simulink model "BPSK"  (R2024b)
settings: Solver=VariableStepAuto  StartTime=0.0  StopTime=10.0  RelTol=1e-3
undefined symbols (not defined in the file or in its folder): comm, constellation
libraries: commdigbbndpm3 x2, commchan3 x1, commutil2 x1, commsink2 x1, commrflib2 x1, commrandsrc3 x1
settings Model: Creator=sarriola  LastModifiedBy=romaf41
settings SolverCC: AlgebraicLoopSolver=TrustRegion
settings DataIOCC: ReturnWorkspaceOutputs=off
settings DebuggingCC: UnconnectedInputMsg=warning  UnconnectedOutputMsg=warning  UnconnectedLineMsg=warning  ArithmeticOperatorsInVariantConditions=warning
settings ModelReferenceCC: EnableRefExpFcnMdlSchedulingChecks=on
settings SFSimCC: SimUseLocalCustomCode=off  CustomCodeUndefinedFunction=UseInterfaceOnly
settings RTWCC: RTWUseLocalCustomCode=off  GPUComputeCapability=3.5
settings CodeAppCC: StateflowObjectComments=on

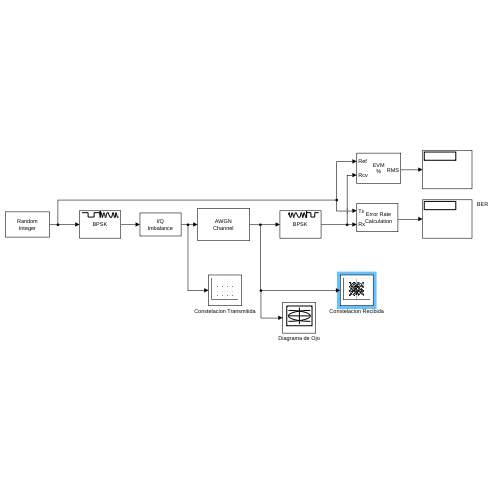
[thumbnail: Simulink's stored preview of the top-level diagram]
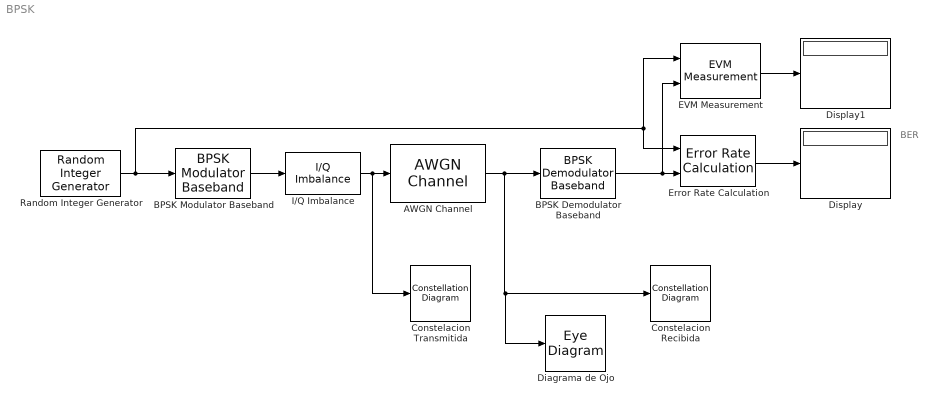
== system BPSK ==
  note: BER
  AWGN Channel : commchan3/AWGN Channel  LegacyMode=on  NoiseMethod="Signal to noise ratio  (SNR)"  noiseMode="Signal to noise ratio  (SNR)"  EbNo=10  EsNo=10  SNR=10  BitsPerSymbol=3  SignalPower=1  SamplesPerSymbol=1  SymbolPeriod=1e-6  VarianceSource=Parameter  Variance=1  RandomStream=Global stream  Seed=67  SimulateUsing=Code generation
  BPSK Demodulator Baseband : commdigbbndpm3/BPSK Demodulator Baseband  DecType=Hard decision  VarSource=Dialog  Variance=1  Ph=0  outDtype=Inherit via internal rule  derotateFactorWordLen=16  derotateFactorDataTypeStr=Inherit: Same word length as input  derotateFactorLastDataTypeStr=Inherit: Same word length as input
  BPSK Modulator Baseband : commdigbbndpm3/BPSK Modulator Baseband  Ph=0  outDtype=double  outWordLen=16  outUDDataType=sfix(16)  outFracLenMode=Best precision  outFracLen=15  outDataTypeStr=double  outLastDataTypeStr=double
  "Constelacion Recibida " : ConstellationDiagram  WindowPosition=[-95 -36 1366 640]  ReferenceConstellation=BPSK  ShowTrajectory=on  EnableMeasurements=on  DefaultConfigurationName=comm.scopes.ConstellationDiagramBlockCfg
  Constelacion Transmitida : ConstellationDiagram  WindowPosition=[-597 -97 1370 695]  ShowTrajectory=on  DefaultConfigurationName=comm.scopes.ConstellationDiagramBlockCfg
  "Diagrama de Ojo " : EyeDiagram
  Display : Display
  Display1 : Display
  EVM Measurement : commutil2/EVM Measurement  Normalization=Average reference signal power  AverageConstellationPower=1  PeakConstellationPower=1  ReferenceSignalSource=Input port  ReferenceConstellation=constellation( comm.QPSKModulator )  MeasurementIntervalSource=Input length  MeasurementInterval=100  AveragingDimensions=1  MaximumEVMOutputPort=off  XPercentileEVMOutputPort=off  XPercentileValue=95  SymbolCountOutputPort=off  SimulateUsing=Interpreted execution
  Error Rate Calculation : commsink2/Error Rate Calculation  N=0  st_delay=0  cp_mode=Entire frame  subframe=[]  PMode=Port  WsName=ErrorVec  RsMode2=off  stop=off  numErr=100  maxBits=1e6
  I/Q Imbalance : commrflib2/I//Q Imbalance  ampImbal=-10  phsImbal=45  Idc=0  Qdc=0
  Random Integer Generator : commrandsrc3/Random Integer Generator  SetSize=2  SeedSource=Auto  Seed=0  SampleTime=1e-6  SamplesPerFrame=1024  OutputDataType=double  SimulateUsing=Interpreted execution
  wires:
  EVM Measurement/1 -> Display1/1
  AWGN Channel/1 -> BPSK Demodulator Baseband/1, "Diagrama de Ojo "/1, "Constelacion Recibida "/1
  Error Rate Calculation/1 -> Display/1
  BPSK Demodulator Baseband/1 -> EVM Measurement/2, Error Rate Calculation/2
  Random Integer Generator/1 -> BPSK Modulator Baseband/1, EVM Measurement/1, Error Rate Calculation/1
  BPSK Modulator Baseband/1 -> I/Q Imbalance/1
  I/Q Imbalance/1 -> Constelacion Transmitida/1, AWGN Channel/1
